simulink model "pid_ff_design_final"  (R2019b)
settings: Solver=FixedStepAuto  StartTime=0.0  StopTime=4  FixedStep=0.001  RelTol=1e-3
settings Model: Creator=subhgang  LastModifiedBy=subhgang

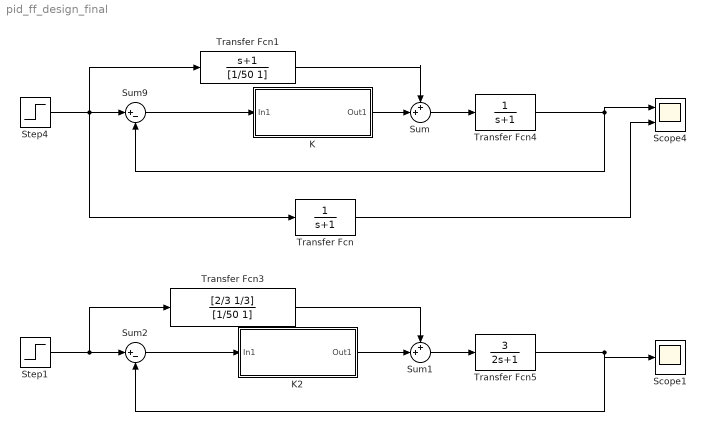
== system pid_ff_design_final ==
  K : Subsystem
  K2 : Subsystem
  Scope1 : Scope
  Scope4 : Scope  NumInputPorts=2
  Step1 : Step  SampleTime=0
  Step4 : Step  SampleTime=0
  Sum : Sum  Inputs=++|
  Sum1 : Sum  Inputs=++|
  Sum2 : Sum  Inputs=|+-
  Sum9 : Sum  Inputs=|+-
  Transfer Fcn : TransferFcn  Denominator=[1 1]
  Transfer Fcn1 : TransferFcn  Numerator=[1 1]  Denominator=[1/50 1]
  Transfer Fcn3 : TransferFcn  Numerator=[2/3 1/3]  Denominator=[1/50 1]
  Transfer Fcn4 : TransferFcn  Denominator=[1 1]
  Transfer Fcn5 : TransferFcn  Numerator=[3]  Denominator=[2 1]
  wires:
  Sum9/1 -> K/1(In1)
  Transfer Fcn4/1 -> Scope4/1, Sum9/2
  Transfer Fcn/1 -> Scope4/2
  Step4/1 -> Transfer Fcn1/1, Transfer Fcn/1, Sum9/1
  Transfer Fcn1/1 -> Sum/1
  Sum/1 -> Transfer Fcn4/1
  K/1(Out1) -> Sum/2
  Transfer Fcn5/1 -> Scope1/1, Sum2/2
  Sum2/1 -> K2/1(In1)
  Step1/1 -> Transfer Fcn3/1, Sum2/1
  K2/1(Out1) -> Sum1/2
  Sum1/1 -> Transfer Fcn5/1
  Transfer Fcn3/1 -> Sum1/1

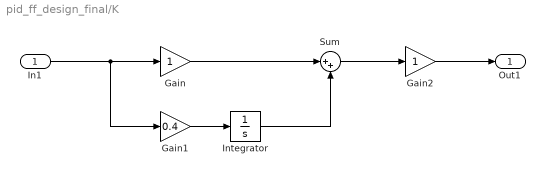
== system pid_ff_design_final/K ==
  In1 : Inport
  Gain : Gain
  Gain1 : Gain  Gain=0.4
  Gain2 : Gain
  Integrator : Integrator
  Sum : Sum  Inputs=|++
  Out1 : Outport
  wires:
  In1/1 -> Gain1/1, Gain/1
  Gain1/1 -> Integrator/1
  Gain/1 -> Sum/1
  Integrator/1 -> Sum/2
  Sum/1 -> Gain2/1
  Gain2/1 -> Out1/1

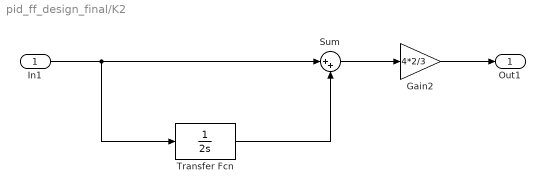
== system pid_ff_design_final/K2 ==
  In1 : Inport
  Gain2 : Gain  Gain=4*2/3
  Sum : Sum  Inputs=|++
  Transfer Fcn : TransferFcn  Denominator=[2 0]
  Out1 : Outport
  wires:
  In1/1 -> Transfer Fcn/1, Sum/1
  Sum/1 -> Gain2/1
  Gain2/1 -> Out1/1
  Transfer Fcn/1 -> Sum/2
